simulink model "IBVSstereo"  (Simulink 5.0)
settings: Solver=ode45  StartTime=0.0  StopTime=30.0  RelTol=1e-3
values from neighbouring files (symbols this model uses):
  lc =     [task_stereo.mat]
  p = reshape(u,2,n)    [CamView.m]    (also in initHBVS.m = polyhedra([0.0 0.0 0; 0.25 0.25 0; -0.25 0.25 0; -0.25 -0.25; pose0.mat = ; pose1.mat = ; sim1.mat = )
  rc =     [task_stereo.mat]
  T0e_0 =     [task_endeff.mat]    (also in task_stereo.mat)
  T0e_x =     [task_endeff.mat]    (also in task_stereo.mat)
  T0o =     [pose0.mat]    (also in pose1.mat; sim1.mat; task_endeff.mat; task_stereo.mat)
  Telc =     [task_stereo.mat]
  Terc =     [task_stereo.mat]
undefined symbols (not defined in the file or in its folder): coords, get, GetHMatrix
libraries: vs x31, simulink x3
settings Model: LastModifiedBy=ecervera  BooleanDataType=off

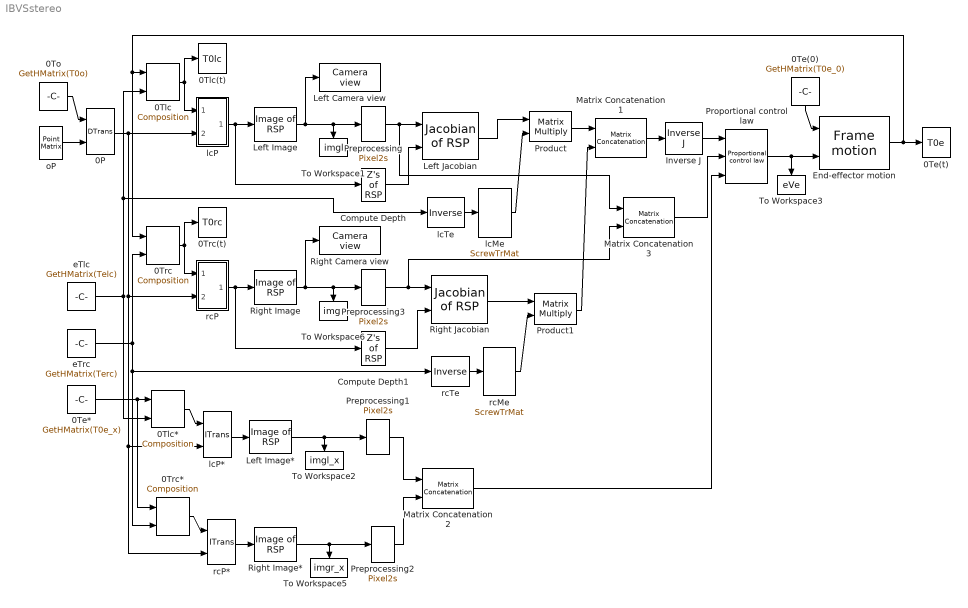
== system IBVSstereo ==
  0P : vs/Features/DTrans  SimViewingDevice=off  DataTypeOverride=UseLocalSettings  MinMaxOverflowLogging=UseLocalSettings
      settings: Permissions=ReadWrite  RTWFcnNameOpts=Auto  RTWFileNameOpts=Auto
  0Te(0) : Constant  Orientation=down  Value=GetHMatrix(T0e_0)  VectorParams1D=off
  0Te(t) : ToWorkspace  VariableName=T0e  SampleTime=-1  SaveFormat=StructureWithTime
  0Te* : Constant  Value=GetHMatrix(T0e_x)  VectorParams1D=off
  0Tlc : vs/Pose/Composition  SimViewingDevice=off  DataTypeOverride=UseLocalSettings  MinMaxOverflowLogging=UseLocalSettings
      settings: Permissions=ReadWrite  RTWFcnNameOpts=Auto  RTWFileNameOpts=Auto
  0Tlc(t) : ToWorkspace  VariableName=T0lc  SampleTime=-1  SaveFormat=StructureWithTime
  0Tlc* : vs/Pose/Composition  SimViewingDevice=off  DataTypeOverride=UseLocalSettings  MinMaxOverflowLogging=UseLocalSettings
      settings: Permissions=ReadWrite  RTWFcnNameOpts=Auto  RTWFileNameOpts=Auto
  0To : Constant  Value=GetHMatrix(T0o)  VectorParams1D=off
  0Trc : vs/Pose/Composition  SimViewingDevice=off  DataTypeOverride=UseLocalSettings  MinMaxOverflowLogging=UseLocalSettings
      settings: Permissions=ReadWrite  RTWFcnNameOpts=Auto  RTWFileNameOpts=Auto
  0Trc(t) : ToWorkspace  VariableName=T0rc  SampleTime=-1  SaveFormat=StructureWithTime
  0Trc* : vs/Pose/Composition  SimViewingDevice=off  DataTypeOverride=UseLocalSettings  MinMaxOverflowLogging=UseLocalSettings
      settings: Permissions=ReadWrite  RTWFcnNameOpts=Auto  RTWFileNameOpts=Auto
  Compute Depth : vs/Features/Z's of RSP  SimViewingDevice=off  DataTypeOverride=UseLocalSettings  MinMaxOverflowLogging=UseLocalSettings
      settings: Permissions=ReadWrite  RTWFcnNameOpts=Auto  RTWFileNameOpts=Auto
  Compute Depth1 : vs/Features/Z's of RSP  SimViewingDevice=off  DataTypeOverride=UseLocalSettings  MinMaxOverflowLogging=UseLocalSettings
      settings: Permissions=ReadWrite  RTWFcnNameOpts=Auto  RTWFileNameOpts=Auto
  End-effector motion : vs/Pose/Frame motion  SimViewingDevice=off  DataTypeOverride=UseLocalSettings  MinMaxOverflowLogging=UseLocalSettings
      settings: Permissions=ReadWrite  RTWFcnNameOpts=Auto  RTWFileNameOpts=Auto
  Inverse J : vs/Jacobian/Inverse J  SimViewingDevice=off  DataTypeOverride=UseLocalSettings  MinMaxOverflowLogging=UseLocalSettings
      settings: Permissions=ReadWrite  RTWFcnNameOpts=Auto  RTWFileNameOpts=Auto
  Left Camera view : vs/Camera/Camera view  ms=15  em=normal  umin=0  umax=get(lc,'hres')-1  vmin=0  vmax=get(lc,'vres')-1  st=-1
  Left Image : vs/Camera/Image of RSP  fu=get(lc,'fu')  fv=get(lc,'fv')  u0=get(lc,'u0')  v0=get(lc,'v0')
  Left Image* : vs/Camera/Image of RSP  fu=get(lc,'fu')  fv=get(lc,'fv')  u0=get(lc,'u0')  v0=get(lc,'v0')
  Left Jacobian : vs/Jacobian/Jacobian of RSP  SimViewingDevice=off  DataTypeOverride=UseLocalSettings  MinMaxOverflowLogging=UseLocalSettings
      settings: Permissions=ReadWrite  RTWFcnNameOpts=Auto  RTWFileNameOpts=Auto
  Matrix Concatenation1 : simulink/Math Operations/Matrix Concatenation  numInports=2  catMethod=Vertical
  Matrix Concatenation2 : simulink/Math Operations/Matrix Concatenation  numInports=2  catMethod=Vertical
  Matrix Concatenation3 : simulink/Math Operations/Matrix Concatenation  numInports=2  catMethod=Vertical
  Preprocessing : vs/Jacobian/Pixel2s  fu=get(lc,'fu')  fv=get(lc,'fv')  u0=get(lc,'u0')  v0=get(lc,'v0')
  Preprocessing1 : vs/Jacobian/Pixel2s  fu=get(lc,'fu')  fv=get(lc,'fv')  u0=get(lc,'u0')  v0=get(lc,'v0')
  Preprocessing2 : vs/Jacobian/Pixel2s  fu=get(rc,'fu')  fv=get(rc,'fv')  u0=get(rc,'u0')  v0=get(rc,'v0')
  Preprocessing3 : vs/Jacobian/Pixel2s  fu=get(rc,'fu')  fv=get(rc,'fv')  u0=get(rc,'u0')  v0=get(rc,'v0')
  Product : Product  Multiplication=Matrix(*)  SaturateOnIntegerOverflow=on  InputSameDT=on
  Product1 : Product  Multiplication=Matrix(*)  SaturateOnIntegerOverflow=on  InputSameDT=on
  Proportional control law : vs/Jacobian/Proportional control law  lambda=lambda
  Right Camera view : vs/Camera/Camera view  ms=15  em=normal  umin=0  umax=get(rc,'hres')-1  vmin=0  vmax=get(rc,'vres')-1  st=-1
  Right Image : vs/Camera/Image of RSP  fu=get(rc,'fu')  fv=get(rc,'fv')  u0=get(rc,'u0')  v0=get(rc,'v0')
  Right Image* : vs/Camera/Image of RSP  fu=get(rc,'fu')  fv=get(rc,'fv')  u0=get(rc,'u0')  v0=get(rc,'v0')
  Right Jacobian : vs/Jacobian/Jacobian of RSP  SimViewingDevice=off  DataTypeOverride=UseLocalSettings  MinMaxOverflowLogging=UseLocalSettings
      settings: Permissions=ReadWrite  RTWFcnNameOpts=Auto  RTWFileNameOpts=Auto
  To Workspace1 : ToWorkspace  VariableName=imgl  SampleTime=-1  SaveFormat=StructureWithTime
      settings: Orientation=down
  To Workspace2 : ToWorkspace  VariableName=imgl_x  SampleTime=-1  SaveFormat=StructureWithTime
      settings: Orientation=down
  To Workspace3 : ToWorkspace  VariableName=eVe  SampleTime=-1  SaveFormat=StructureWithTime
      settings: Orientation=down
  To Workspace5 : ToWorkspace  VariableName=imgr_x  SampleTime=-1  SaveFormat=StructureWithTime
      settings: Orientation=down
  To Workspace6 : ToWorkspace  VariableName=imgr  SampleTime=-1  SaveFormat=StructureWithTime
      settings: Orientation=down
  eTlc : Constant  Value=GetHMatrix(Telc)  VectorParams1D=off
  eTrc : Constant  Value=GetHMatrix(Terc)  VectorParams1D=off
  lcMe : vs/Pose/ScrewTrMat  SimViewingDevice=off  DataTypeOverride=UseLocalSettings  MinMaxOverflowLogging=UseLocalSettings
      settings: Permissions=ReadWrite  RTWFcnNameOpts=Auto  RTWFileNameOpts=Auto
  lcP : Subsystem  AncestorBlock=vs/Features/ITrans
  lcP* : vs/Features/ITrans  SimViewingDevice=off  DataTypeOverride=UseLocalSettings  MinMaxOverflowLogging=UseLocalSettings
      settings: Permissions=ReadWrite  RTWFcnNameOpts=Auto  RTWFileNameOpts=Auto
  lcTe : vs/Pose/Inverse  SimViewingDevice=off  DataTypeOverride=UseLocalSettings  MinMaxOverflowLogging=UseLocalSettings
      settings: Permissions=ReadWrite  RTWFcnNameOpts=Auto  RTWFileNameOpts=Auto
  oP : vs/Features/Point Matrix  m=coords(p)
  rcMe : vs/Pose/ScrewTrMat  SimViewingDevice=off  DataTypeOverride=UseLocalSettings  MinMaxOverflowLogging=UseLocalSettings
      settings: Permissions=ReadWrite  RTWFcnNameOpts=Auto  RTWFileNameOpts=Auto
  rcP : Subsystem  AncestorBlock=vs/Features/ITrans
  rcP* : vs/Features/ITrans  SimViewingDevice=off  DataTypeOverride=UseLocalSettings  MinMaxOverflowLogging=UseLocalSettings
      settings: Permissions=ReadWrite  RTWFcnNameOpts=Auto  RTWFileNameOpts=Auto
  rcTe : vs/Pose/Inverse  SimViewingDevice=off  DataTypeOverride=UseLocalSettings  MinMaxOverflowLogging=UseLocalSettings
      settings: Permissions=ReadWrite  RTWFcnNameOpts=Auto  RTWFileNameOpts=Auto
  wires:
  oP/1 -> 0P/2
  lcP/1(bP) -> Compute Depth/1, Left Image/1
  Left Image/1 -> Left Camera view/1, Preprocessing/1, To Workspace1/1
  Preprocessing/1 -> Left Jacobian/1, Matrix Concatenation3/1
  Compute Depth/1 -> Left Jacobian/2
  Inverse J/1 -> Proportional control law/1
  End-effector motion/1 -> 0Te(t)/1, 0Tlc/1, 0Trc/1
  0Te*/1 -> 0Tlc*/1, 0Trc*/1
  lcP*/1 -> Left Image*/1
  0Te(0)/1 -> End-effector motion/1
  0To/1 -> 0P/1
  0P/1 -> lcP/2(aP), lcP*/2, rcP*/2, rcP/2(aP)
  Proportional control law/1 -> End-effector motion/2, To Workspace3/1
  Left Image*/1 -> Preprocessing1/1, To Workspace2/1
  0Tlc/1 -> lcP/1(aTb), 0Tlc(t)/1
  eTlc/1 -> 0Tlc*/2, 0Tlc/2, lcTe/1
  0Tlc*/1 -> lcP*/1
  rcP*/1 -> Right Image*/1
  Right Image*/1 -> Preprocessing2/1, To Workspace5/1
  0Trc*/1 -> rcP*/1
  eTrc/1 -> 0Trc/2, 0Trc*/2, rcTe/1
  rcP/1(bP) -> Compute Depth1/1, Right Image/1
  Right Image/1 -> Right Camera view/1, Preprocessing3/1, To Workspace6/1
  Preprocessing3/1 -> Right Jacobian/1, Matrix Concatenation3/2
  Compute Depth1/1 -> Right Jacobian/2
  0Trc/1 -> rcP/1(aTb), 0Trc(t)/1
  lcTe/1 -> lcMe/1
  Product/1 -> Matrix Concatenation1/1
  Matrix Concatenation1/1 -> Inverse J/1
  Left Jacobian/1 -> Product/1
  lcMe/1 -> Product/2
  rcTe/1 -> rcMe/1
  rcMe/1 -> Product1/2
  Right Jacobian/1 -> Product1/1
  Product1/1 -> Matrix Concatenation1/2
  Preprocessing1/1 -> Matrix Concatenation2/1
  Preprocessing2/1 -> Matrix Concatenation2/2
  Matrix Concatenation3/1 -> Proportional control law/2
  Matrix Concatenation2/1 -> Proportional control law/3

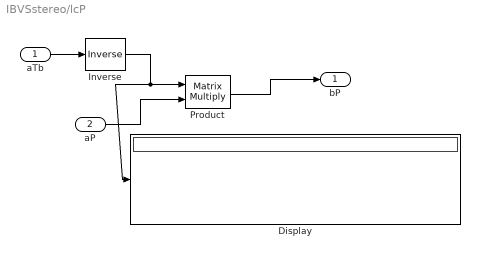
== system IBVSstereo/lcP ==
  aTb : Inport
  aP : Inport  Port=2
  Display : Display
  Inverse : vs/Pose/Inverse  SimViewingDevice=off  DataTypeOverride=UseLocalSettings  MinMaxOverflowLogging=UseLocalSettings
      settings: Permissions=ReadWrite  RTWFcnNameOpts=Auto  RTWFileNameOpts=Auto
  Product : Product  Multiplication=Matrix(*)  SaturateOnIntegerOverflow=on  InputSameDT=on
  bP : Outport
  wires:
  Inverse/1 -> Product/1, Display/1
  aTb/1 -> Inverse/1
  Product/1 -> bP/1
  aP/1 -> Product/2

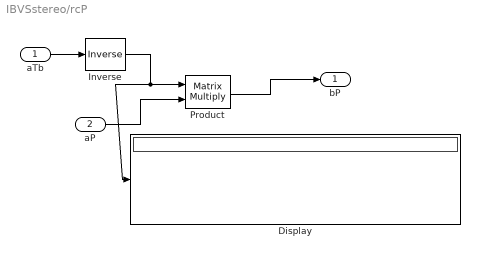
== system IBVSstereo/rcP ==
  aTb : Inport
  aP : Inport  Port=2
  Display : Display
  Inverse : vs/Pose/Inverse  SimViewingDevice=off  DataTypeOverride=UseLocalSettings  MinMaxOverflowLogging=UseLocalSettings
      settings: Permissions=ReadWrite  RTWFcnNameOpts=Auto  RTWFileNameOpts=Auto
  Product : Product  Multiplication=Matrix(*)  SaturateOnIntegerOverflow=on  InputSameDT=on
  bP : Outport
  wires:
  Inverse/1 -> Product/1, Display/1
  aTb/1 -> Inverse/1
  Product/1 -> bP/1
  aP/1 -> Product/2
